simulink model "A_ZH_Z3"  (R2025a)
settings: Solver=VariableStepAuto  StartTime=0.0  StopTime=10  RelTol=1e-3
settings Model: Creator=Szalay  LastModifiedBy=Szalay

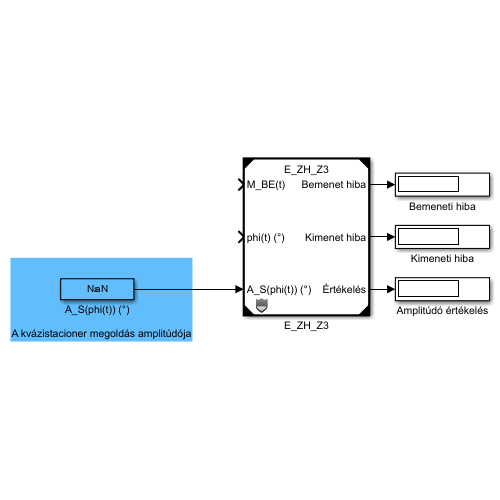
[thumbnail: Simulink's stored preview of the top-level diagram]
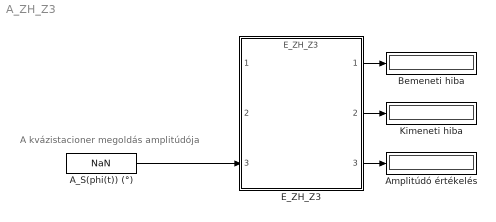
== system A_ZH_Z3 ==
  note: A kvázistacioner megoldás amplitúdója
  A_S(phi(t)) (°) : Constant  Value=NaN
  Amplitúdó értékelés : Display
  Bemeneti hiba : Display
  E_ZH_Z3 : ModelReference  ModelNameDialog=E_ZH_Z3.slxp  ModelReferenceVersion=1.15  CopyOfModelProtected=on
  Kimeneti hiba : Display
  wires:
  E_ZH_Z3/1 -> Bemeneti hiba/1
  E_ZH_Z3/2 -> Kimeneti hiba/1
  A_S(phi(t)) (°)/1 -> E_ZH_Z3/3
  E_ZH_Z3/3 -> Amplitúdó értékelés/1
